simulink model "Bioloid_HIK_mdl"  (R2013a)
settings: Solver=ode1  StartTime=0  StopTime=inf  FixedStep=0.01  RelTol=1e-3
undefined symbols (not defined in the file or in its folder): Bioloid_HIK, Bioloid_Signals2VRML
libraries: vrlib x1
settings Model: Creator=root  LastModifiedBy=root

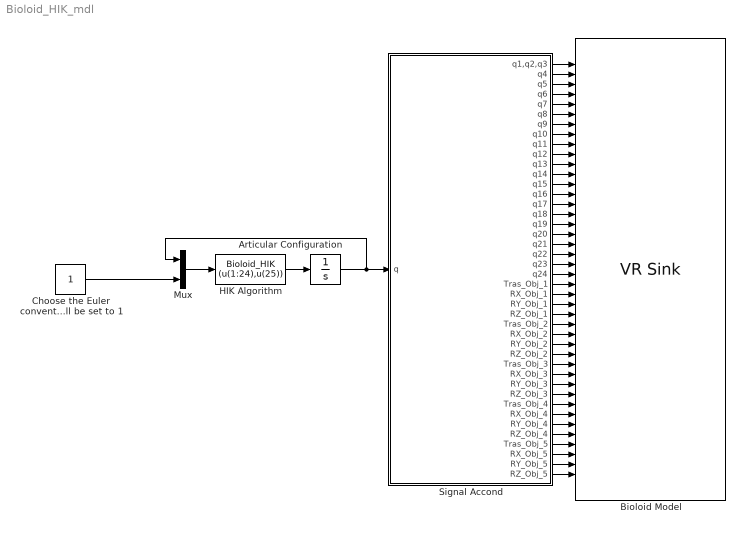
== system Bioloid_HIK_mdl ==
  Articular Configuration : Integrator
  Bioloid Model : vrlib/VR Sink  InstantiateOnLoad=on  SampleTime=0.1  ViewEnable=on  RemoteChange=off  RemoteView=off  FieldsWritten=TrunkTraslation.translation.3.1.1.double#TrunkRotX.rotation.4.1.1.double#TrunkRotY.rotation.4.1.1.double#TrunkRotZ.rotation.4.1.1.double#Right_Arm.rotation.4.1.1.double#Right_Humeros1.rotation.4.1.1.double#Right_Hand1.rotation.4.1.1.double#Left_Arm.rotation.4.1.1.double#Left_Humeros1.rotation.4.1.1.double#Left_Hand1.rotation.4.1.1.double#Right_Groin.rotation.4.1.1.double#Right_Hip1.rotation.4.1.1.double#Right_Femur1.rotation.4.1.1.double#Right_Tibia1.rotation.4.1.1.double#Right_Ankle1.rotation.4.1.1.double#Right_Foot1.rotation.4.1.1.double#Left_Groin.rotation.4.1.1.double#Left_Hip1.rotation.4.1.1.double#Left_Femur1.rotation.4.1.1.double#Left_Tibia1.rotation.4.1.1.double#Left_Ankle1.rotation.4.1.1.double#Left_Foot1.rotation.4.1.1.double#Obj_1_Tras.translation.3.1.1.double#Obj_1_RotX.rotation.4.1.1.double#Obj_1_RotY.rotation.4.1.1.double#Obj_1_RotZ.rotation.4.1.1.double#Obj_2_Tras.translation.3.1.1.double#Obj_2_RotX.rotation.4.1.1.double#Obj_2_RotY.rotation.4.1.1.double#Obj_2_RotZ.rotation.4.1.1.double#Obj_3_Tras.translation.3.1.1.double#Obj_3_RotX.rotation.4.1.1.double#Obj_3_RotY.rotation.4.1.1.double#Obj_3_RotZ.rotation.4.1.1.double#Obj_4_Tras.translation.3.1.1.double#Obj_4_RotX.rotation.4.1.1.double#Obj_4_RotY.rotation.4.1.1.double#Obj_4_RotZ.rotation.4.1.1.double#Obj_5_Tras.translation.3.1.1.double#Obj_5_RotX.rotation.4.1.1.double#Obj_5_RotY.rotation.4.1.1.double#Obj_5_RotZ.rotation.4.1.1.double  WorldFileName=Bioloid_model_5_obj.wrl  WorldDescription=Bioloid Model for HIK  AutoView=on  VideoDimensions=[]  AllowVariableSize=off  FigureProperties="{'Position', 'Name', 'Viewpoint', 'CameraBound', 'CameraDirection', 'CameraPosition', 'CameraUpVector', 'ZoomFactor', 'Antialiasing', 'Headlight', 'Lighting', 'NavPanel', 'StatusBar', 'ToolBar', 'Textures', 'Transparency', 'Triad', 'Wireframe', 'NavZones', 'NavMode', 'NavSpeed', 'CaptureFileFormat', 'CaptureFileName', 'Record2DCompressMethod', 'Record2DCompressQuality', 'Record2D', 'Record2DFileName', 'Record2DFPS'; [6.6000000000000000e+01   7.8000000000000000e+01   1.3010000000000000e+03   6.3900000000000000e+02], 'Bioloid Model for HIK', '_untitled_12', 'on', [0.0000000000000000e+00   4.9979169270678366e-02  -9.9875026039496628e-01], [0.0000000000000000e+00   0.0000000000000000e+00   0.0000000000000000e+00], [0.0000000000000000e+00   9.9875026039496628e-01   4.9979169270678366e-02], [1.0000000000000000e+00], 'on', 'on', 'on', 'halfbar', 'on', 'on', 'on', 'on', 'none', 'off', 'off', 'fly', 'normal', 'tif', '%f_anim_%n.tif', 'auto', [7.5000000000000000e+01], 'on', '%f_anim_%n.avi', [1.5000000000000000e+01]}"
  Choose the Euler convention 1.- XYZ 2.- XZY 3.- XYX 4.- XZX 5.- YXZ 6.- YZX 7.- YXY 8.- YZY 9.- ZXY 10.- ZYX 11.- ZXZ 12.- ZYZ if any other is chosen it will be set to 1 : Constant
  HIK Algorithm : MATLABFcn  MATLABFcn=Bioloid_HIK (u(1:24),u(25))  OutputDimensions=24
  Mux : Mux  Inputs=2
  Signal Accond : Subsystem
  wires:
  Choose the Euler convention 1.- XYZ 2.- XZY 3.- XYX 4.- XZX 5.- YXZ 6.- YZX 7.- YXY 8.- YZY 9.- ZXY 10.- ZYX 11.- ZXZ 12.- ZYZ if any other is chosen it will be set to 1/1 -> Mux/2
  Mux/1 -> HIK Algorithm/1
  HIK Algorithm/1 -> Articular Configuration/1
  Articular Configuration/1 -> Signal Accond/1(q), Mux/1
  Signal Accond/29(RY_Obj_2) -> Bioloid Model/29
  Signal Accond/32(RX_Obj_3) -> Bioloid Model/32
  Signal Accond/26(RZ_Obj_1) -> Bioloid Model/26
  Signal Accond/42(RZ_Obj_5) -> Bioloid Model/42
  Signal Accond/36(RX_Obj_4) -> Bioloid Model/36
  Signal Accond/27(Tras_Obj_2) -> Bioloid Model/27
  Signal Accond/39(Tras_Obj_5) -> Bioloid Model/39
  Signal Accond/41(RY_Obj_5) -> Bioloid Model/41
  Signal Accond/30(RZ_Obj_2) -> Bioloid Model/30
  Signal Accond/34(RZ_Obj_3) -> Bioloid Model/34
  Signal Accond/28(RX_Obj_2) -> Bioloid Model/28
  Signal Accond/22(q24) -> Bioloid Model/22
  Signal Accond/35(Tras_Obj_4) -> Bioloid Model/35
  Signal Accond/18(q20) -> Bioloid Model/18
  Signal Accond/31(Tras_Obj_3) -> Bioloid Model/31
  Signal Accond/2(q4) -> Bioloid Model/2
  Signal Accond/10(q12) -> Bioloid Model/10
  Signal Accond/3(q5) -> Bioloid Model/3
  Signal Accond/4(q6) -> Bioloid Model/4
  Signal Accond/19(q21) -> Bioloid Model/19
  Signal Accond/11(q13) -> Bioloid Model/11
  Signal Accond/5(q7) -> Bioloid Model/5
  Signal Accond/6(q8) -> Bioloid Model/6
  Signal Accond/7(q9) -> Bioloid Model/7
  Signal Accond/8(q10) -> Bioloid Model/8
  Signal Accond/9(q11) -> Bioloid Model/9
  Signal Accond/37(RY_Obj_4) -> Bioloid Model/37
  Signal Accond/33(RY_Obj_3) -> Bioloid Model/33
  Signal Accond/12(q14) -> Bioloid Model/12
  Signal Accond/13(q15) -> Bioloid Model/13
  Signal Accond/23(Tras_Obj_1) -> Bioloid Model/23
  Signal Accond/21(q23) -> Bioloid Model/21
  Signal Accond/24(RX_Obj_1) -> Bioloid Model/24
  Signal Accond/14(q16) -> Bioloid Model/14
  Signal Accond/17(q19) -> Bioloid Model/17
  Signal Accond/15(q17) -> Bioloid Model/15
  Signal Accond/16(q18) -> Bioloid Model/16
  Signal Accond/25(RY_Obj_1) -> Bioloid Model/25
  Signal Accond/20(q22) -> Bioloid Model/20
  Signal Accond/38(RZ_Obj_4) -> Bioloid Model/38
  Signal Accond/40(RX_Obj_5) -> Bioloid Model/40
  Signal Accond/1(q1,q2,q3) -> Bioloid Model/1

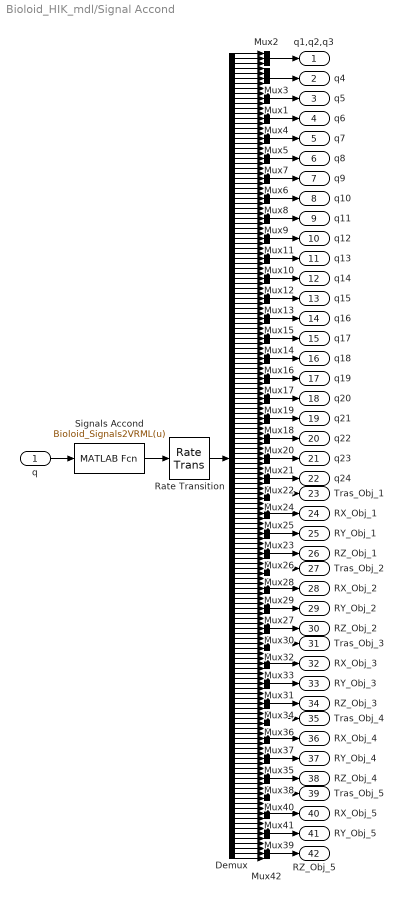
== system Bioloid_HIK_mdl/Signal Accond ==
  q : Inport
  Demux : Demux  Outputs=162
  Mux{1,3..23,25..27,29..31,33..35,37..39,41..42} (36 alike) : Mux
  Mux{2,24,28,32,36,40} (6 alike) : Mux  Inputs=3
  Rate Transition : RateTransition  OutPortSampleTime=0.1
  "Signals Accond " : MATLABFcn  MATLABFcn=Bioloid_Signals2VRML(u)  OutputDimensions=162
  q1,q2,q3 : Outport
  q4 : Outport  Port=2
  q5 : Outport  Port=3
  q6 : Outport  Port=4
  q7 : Outport  Port=5
  q8 : Outport  Port=6
  q9 : Outport  Port=7
  q10 : Outport  Port=8
  q11 : Outport  Port=9
  q12 : Outport  Port=10
  q13 : Outport  Port=11
  q14 : Outport  Port=12
  q15 : Outport  Port=13
  q16 : Outport  Port=14
  q17 : Outport  Port=15
  q18 : Outport  Port=16
  q19 : Outport  Port=17
  q20 : Outport  Port=18
  q21 : Outport  Port=19
  q22 : Outport  Port=20
  q23 : Outport  Port=21
  q24 : Outport  Port=22
  Tras_Obj_1 : Outport  Port=23
  RX_Obj_1 : Outport  Port=24
  RY_Obj_1 : Outport  Port=25
  RZ_Obj_1 : Outport  Port=26
  Tras_Obj_2 : Outport  Port=27
  RX_Obj_2 : Outport  Port=28
  RY_Obj_2 : Outport  Port=29
  RZ_Obj_2 : Outport  Port=30
  Tras_Obj_3 : Outport  Port=31
  RX_Obj_3 : Outport  Port=32
  RY_Obj_3 : Outport  Port=33
  RZ_Obj_3 : Outport  Port=34
  Tras_Obj_4 : Outport  Port=35
  RX_Obj_4 : Outport  Port=36
  RY_Obj_4 : Outport  Port=37
  RZ_Obj_4 : Outport  Port=38
  Tras_Obj_5 : Outport  Port=39
  RX_Obj_5 : Outport  Port=40
  RY_Obj_5 : Outport  Port=41
  RZ_Obj_5 : Outport  Port=42
  wires:
  q/1 -> "Signals Accond "/1
  "Signals Accond "/1 -> Rate Transition/1
  Rate Transition/1 -> Demux/1
  Demux/3 -> Mux2/3
  Demux/2 -> Mux2/2
  Demux/1 -> Mux2/1
  Demux/6 -> Mux3/3
  Demux/7 -> Mux3/4
  Demux/4 -> Mux3/1
  Demux/5 -> Mux3/2
  Mux2/1 -> q1,q2,q3/1
  Mux3/1 -> q4/1
  Demux/10 -> Mux1/3
  Demux/11 -> Mux1/4
  Demux/8 -> Mux1/1
  Demux/9 -> Mux1/2
  Mux1/1 -> q5/1
  Demux/14 -> Mux4/3
  Demux/15 -> Mux4/4
  Demux/12 -> Mux4/1
  Demux/13 -> Mux4/2
  Mux4/1 -> q6/1
  Demux/18 -> Mux5/3
  Demux/19 -> Mux5/4
  Demux/16 -> Mux5/1
  Demux/17 -> Mux5/2
  Mux5/1 -> q7/1
  Demux/22 -> Mux7/3
  Demux/23 -> Mux7/4
  Demux/20 -> Mux7/1
  Demux/21 -> Mux7/2
  Mux7/1 -> q8/1
  Demux/26 -> Mux6/3
  Demux/27 -> Mux6/4
  Demux/24 -> Mux6/1
  Demux/25 -> Mux6/2
  Mux6/1 -> q9/1
  Demux/30 -> Mux8/3
  Demux/31 -> Mux8/4
  Demux/28 -> Mux8/1
  Demux/29 -> Mux8/2
  Mux8/1 -> q10/1
  Demux/34 -> Mux9/3
  Demux/35 -> Mux9/4
  Demux/32 -> Mux9/1
  Demux/33 -> Mux9/2
  Mux9/1 -> q11/1
  Demux/38 -> Mux11/3
  Demux/39 -> Mux11/4
  Demux/36 -> Mux11/1
  Demux/37 -> Mux11/2
  Mux11/1 -> q12/1
  Demux/42 -> Mux10/3
  Demux/43 -> Mux10/4
  Demux/40 -> Mux10/1
  Demux/41 -> Mux10/2
  Mux10/1 -> q13/1
  Demux/46 -> Mux12/3
  Demux/47 -> Mux12/4
  Demux/44 -> Mux12/1
  Demux/45 -> Mux12/2
  Mux12/1 -> q14/1
  Demux/50 -> Mux13/3
  Demux/51 -> Mux13/4
  Demux/48 -> Mux13/1
  Demux/49 -> Mux13/2
  Mux13/1 -> q15/1
  Demux/54 -> Mux15/3
  Demux/55 -> Mux15/4
  Demux/52 -> Mux15/1
  Demux/53 -> Mux15/2
  Mux15/1 -> q16/1
  Demux/58 -> Mux14/3
  Demux/59 -> Mux14/4
  Demux/56 -> Mux14/1
  Demux/57 -> Mux14/2
  Mux14/1 -> q17/1
  Demux/62 -> Mux16/3
  Demux/63 -> Mux16/4
  Demux/60 -> Mux16/1
  Demux/61 -> Mux16/2
  Mux16/1 -> q18/1
  Demux/66 -> Mux17/3
  Demux/67 -> Mux17/4
  Demux/64 -> Mux17/1
  Demux/65 -> Mux17/2
  Mux17/1 -> q19/1
  Demux/70 -> Mux19/3
  Demux/71 -> Mux19/4
  Demux/68 -> Mux19/1
  Demux/69 -> Mux19/2
  Mux19/1 -> q20/1
  Demux/74 -> Mux18/3
  Demux/75 -> Mux18/4
  Demux/72 -> Mux18/1
  Demux/73 -> Mux18/2
  Mux18/1 -> q21/1
  Demux/78 -> Mux20/3
  Demux/79 -> Mux20/4
  Demux/76 -> Mux20/1
  Demux/77 -> Mux20/2
  Mux20/1 -> q22/1
  Demux/82 -> Mux21/3
  Demux/83 -> Mux21/4
  Demux/80 -> Mux21/1
  Demux/81 -> Mux21/2
  Mux21/1 -> q23/1
  Mux22/1 -> q24/1
  Demux/84 -> Mux22/1
  Demux/85 -> Mux22/2
  Demux/86 -> Mux22/3
  Demux/87 -> Mux22/4
  Demux/90 -> Mux24/3
  Demux/89 -> Mux24/2
  Demux/88 -> Mux24/1
  Demux/93 -> Mux25/3
  Demux/94 -> Mux25/4
  Demux/91 -> Mux25/1
  Demux/92 -> Mux25/2
  Mux24/1 -> Tras_Obj_1/1
  Mux25/1 -> RX_Obj_1/1
  Demux/97 -> Mux23/3
  Demux/98 -> Mux23/4
  Demux/95 -> Mux23/1
  Demux/96 -> Mux23/2
  Mux23/1 -> RY_Obj_1/1
  Demux/101 -> Mux26/3
  Demux/99 -> Mux26/1
  Demux/100 -> Mux26/2
  Mux26/1 -> RZ_Obj_1/1
  Demux/102 -> Mux26/4
  Demux/105 -> Mux28/3
  Demux/104 -> Mux28/2
  Demux/103 -> Mux28/1
  Demux/108 -> Mux29/3
  Demux/109 -> Mux29/4
  Demux/106 -> Mux29/1
  Demux/107 -> Mux29/2
  Mux28/1 -> Tras_Obj_2/1
  Mux29/1 -> RX_Obj_2/1
  Demux/112 -> Mux27/3
  Demux/113 -> Mux27/4
  Demux/110 -> Mux27/1
  Demux/111 -> Mux27/2
  Mux27/1 -> RY_Obj_2/1
  Demux/116 -> Mux30/3
  Demux/114 -> Mux30/1
  Demux/115 -> Mux30/2
  Mux30/1 -> RZ_Obj_2/1
  Demux/117 -> Mux30/4
  Demux/120 -> Mux32/3
  Demux/119 -> Mux32/2
  Demux/118 -> Mux32/1
  Demux/123 -> Mux33/3
  Demux/124 -> Mux33/4
  Demux/121 -> Mux33/1
  Demux/122 -> Mux33/2
  Mux32/1 -> Tras_Obj_3/1
  Mux33/1 -> RX_Obj_3/1
  Demux/127 -> Mux31/3
  Demux/128 -> Mux31/4
  Demux/125 -> Mux31/1
  Demux/126 -> Mux31/2
  Mux31/1 -> RY_Obj_3/1
  Demux/131 -> Mux34/3
  Demux/129 -> Mux34/1
  Demux/130 -> Mux34/2
  Mux34/1 -> RZ_Obj_3/1
  Demux/132 -> Mux34/4
  Demux/135 -> Mux36/3
  Demux/134 -> Mux36/2
  Demux/133 -> Mux36/1
  Demux/138 -> Mux37/3
  Demux/139 -> Mux37/4
  Demux/136 -> Mux37/1
  Demux/137 -> Mux37/2
  Mux36/1 -> Tras_Obj_4/1
  Mux37/1 -> RX_Obj_4/1
  Demux/142 -> Mux35/3
  Demux/143 -> Mux35/4
  Demux/140 -> Mux35/1
  Demux/141 -> Mux35/2
  Mux35/1 -> RY_Obj_4/1
  Demux/146 -> Mux38/3
  Demux/144 -> Mux38/1
  Demux/145 -> Mux38/2
  Mux38/1 -> RZ_Obj_4/1
  Demux/147 -> Mux38/4
  Demux/150 -> Mux40/3
  Demux/149 -> Mux40/2
  Demux/148 -> Mux40/1
  Demux/153 -> Mux41/3
  Demux/154 -> Mux41/4
  Demux/151 -> Mux41/1
  Demux/152 -> Mux41/2
  Mux40/1 -> Tras_Obj_5/1
  Mux41/1 -> RX_Obj_5/1
  Demux/157 -> Mux39/3
  Demux/158 -> Mux39/4
  Demux/155 -> Mux39/1
  Demux/156 -> Mux39/2
  Mux39/1 -> RY_Obj_5/1
  Demux/161 -> Mux42/3
  Demux/159 -> Mux42/1
  Demux/160 -> Mux42/2
  Mux42/1 -> RZ_Obj_5/1
  Demux/162 -> Mux42/4
